simulink model "mic"  (Simulink 6.6)
libraries: mathlib x26, execlib x7, analoglib x4, genlib x3, arclib x1
settings Model: Creator=Student  LastModifiedBy=REX  MaskType=REX sequence  MaskIconFrame=on  MaskIconOpaque=on  MaskIconRotate=none  MaskIconUnits=autoscale

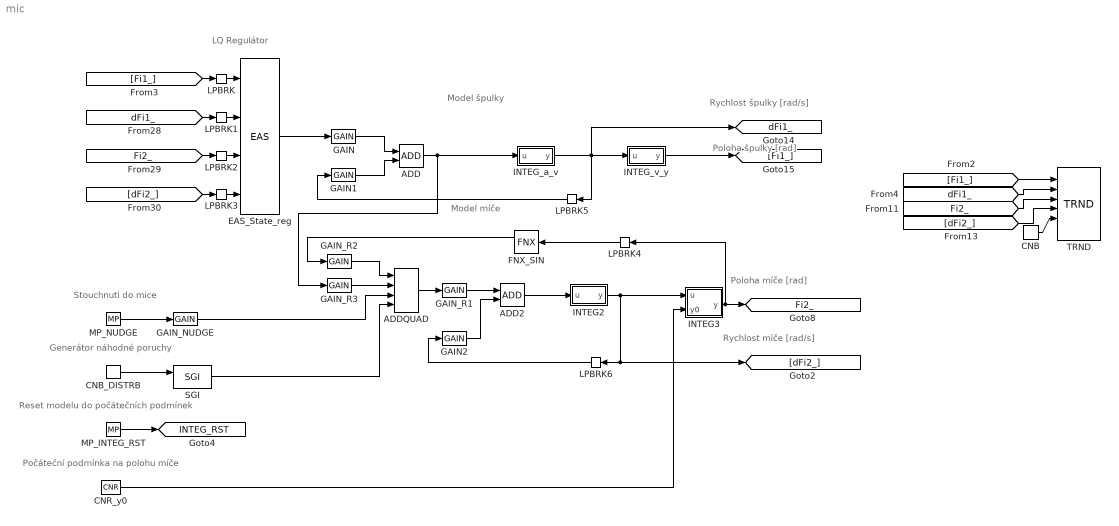
== system mic ==
  note: Stouchnuti do mice
  note: Generátor náhodné poruchy
  note: Reset modelu do počátečních podmínek
  note: Počáteční podmínka na polohu míče
  note: LQ Regulátor
  note: Rychlost špulky [rad/s]
  note: Poloha špulky [rad]
  note: Poloha míče [rad]
  note: Rychlost míče [rad/s]
  note: Model špulky
  note: Model míče
  ADD : mathlib/ADD
  ADD2 : mathlib/ADD
  ADDQUAD : mathlib/ADDQUAD  nl=0
  CNB : mathlib/CNB  SystemSampleTime=-1  YCN=on
  CNB_DISTRB : mathlib/CNB  SystemSampleTime=-1  YCN=on
  CNR_y0 : mathlib/CNR  ycn=0
  EAS_State_reg : mathlib/EAS  a=0.062399  b=1.26032  c=-45.7483  d=-6.60148  y0=0
  FNX_SIN : mathlib/FNX  Orientation=left  ifn=14: sin  yerr=0
  GAIN : mathlib/GAIN  k=85
  GAIN1 : mathlib/GAIN  k=-85
  GAIN2 : mathlib/GAIN  k=-0.3
  GAIN_NUDGE : mathlib/GAIN  k=-0.1
  GAIN_R1 : mathlib/GAIN  k=108.138
  GAIN_R2 : mathlib/GAIN  k=0.3994
  GAIN_R3 : mathlib/GAIN  k=0.0021
  INTEG2 : Subsystem
      mask Type: REX sequence
  INTEG3 : Subsystem
      mask Type: REX sequence
  INTEG_a_v : Subsystem
      mask Type: REX sequence
  INTEG_v_y : Subsystem
      mask Type: REX sequence
  LPBRK{,1..3} (4 alike) : execlib/LPBRK
  LPBRK4 : execlib/LPBRK  Orientation=left
  LPBRK5 : execlib/LPBRK  Orientation=left
  LPBRK6 : execlib/LPBRK  Orientation=left
  MP_INTEG_RST : genlib/MP  BSTATE=off  pwidth=0.5  RPTF=off
  MP_NUDGE : genlib/MP  BSTATE=on  pwidth=0.5  RPTF=off
  SGI : genlib/SGI  isig=4: RANDOM  amp=0.05  freq=1  phase=0  offset=0  ifrunit=1: Hz  iphunit=1: degrees
  TRND : arclib/TRND  SystemSampleTime=-1  n=4  l=10000  btype=8: Double  ptype1=1: Store  ptype2=1: Store  ptype3=1: Store  ptype4=1: Store  pfac=1  afac=0  arc=0  id=1  Title=Ball on spool  timesrc=1  ViewConfig="{\"View\":{\"Data\":{\"History\":20,\"XAxisTimeFormat\":66},\"PropertiesModel\":[{\"Id\":0,\"Items\":[{\"Color\":\"#000099\",\"Id\":0,\"IsActive\":true,\"LineWidth\":2,\"Name\":\"Fi1_\",\"SceneNumber\":1},{\"Color\":\"#669900\",\"Id\":1,\"IsActive\":true,\"LineWidth\":2,\"Name\":\"dFi1_\",\"SceneNumber\":2},{\"Color\":\"#ff0000\",\"Id\":2,\"IsActive\":true,\"LineWidth\":2,\"Name\":\"Fi2_\",\"SceneNumber\":1},{\"Color\":\"#9966cc\",\"Id\":3,\"IsActive\":true,\"LineWidth\":2,\"Name\":\"dFi2_\",\"SceneNumber\":3}]}],\"Scenes\":[{\"Id\":1},{\"Id\":2},{\"Id\":3}],\"sync\":false}}"
  tag scope: Fi2_=global, INTEG_RST=global, dFi1_=global
  wires:
  ADD/1 -> GAIN_R3/1, INTEG_a_v/1(u)
  ADD2/1 -> INTEG2/1(u)
  ADDQUAD/1 -> GAIN_R1/1
  CNB/1 -> TRND/5
  CNB_DISTRB/1 -> SGI/1
  CNR_y0/1 -> INTEG3/2(y0)
  EAS_State_reg/1 -> GAIN/1
  FNX_SIN/1 -> GAIN_R2/1
  [Fi2_] -> TRND/3
  [dFi2_] -> TRND/4
  [Fi1_] -> TRND/1
  [dFi1_] -> LPBRK1/1
  [Fi2_] -> LPBRK2/1
  [Fi1_] -> LPBRK/1
  [dFi2_] -> LPBRK3/1
  [dFi1_] -> TRND/2
  GAIN/1 -> ADD/1
  GAIN1/1 -> ADD/2
  GAIN2/1 -> ADD2/2
  GAIN_NUDGE/1 -> ADDQUAD/3
  GAIN_R1/1 -> ADD2/1
  GAIN_R2/1 -> ADDQUAD/1
  GAIN_R3/1 -> ADDQUAD/2
  INTEG2/1(y) -> [dFi2_], LPBRK6/1, INTEG3/1(u)
  INTEG3/1(y) -> [Fi2_], LPBRK4/1
  INTEG_a_v/1(y) -> [dFi1_], INTEG_v_y/1(u), LPBRK5/1
  INTEG_v_y/1(y) -> [Fi1_]
  LPBRK/1 -> EAS_State_reg/1
  LPBRK1/1 -> EAS_State_reg/2
  LPBRK2/1 -> EAS_State_reg/3
  LPBRK3/1 -> EAS_State_reg/4
  LPBRK4/1 -> FNX_SIN/1
  LPBRK5/1 -> GAIN1/1
  LPBRK6/1 -> GAIN2/1
  MP_INTEG_RST/1 -> [INTEG_RST]
  MP_NUDGE/1 -> GAIN_NUDGE/1
  SGI/1 -> ADDQUAD/4

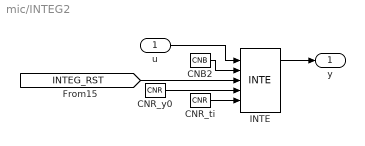
== system mic/INTEG2 ==
  u : Inport  Port=1  OutDataTypeStr=Inherit: auto
  CNB2 : mathlib/CNB  YCN=on
  CNR_ti : mathlib/CNR  ycn=1
  CNR_y0 : mathlib/CNR  ycn=0
  INTE : analoglib/INTE  ymin=-20  ymax=20
  y : Outport  Port=1  OutDataTypeStr=Inherit: auto
  wires:
  CNB2/1 -> INTE/2
  CNR_ti/1 -> INTE/5
  CNR_y0/1 -> INTE/4
  [INTEG_RST] -> INTE/3
  INTE/1 -> y/1
  u/1 -> INTE/1

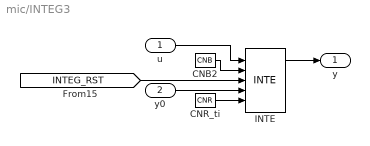
== system mic/INTEG3 ==
  u : Inport  Port=1  OutDataTypeStr=Inherit: auto
  y0 : Inport  Port=2  OutDataTypeStr=Inherit: auto
  CNB2 : mathlib/CNB  YCN=on
  CNR_ti : mathlib/CNR  ycn=1
  INTE : analoglib/INTE  ymin=-0.5  ymax=0.5
  y : Outport  Port=1  OutDataTypeStr=Inherit: auto
  wires:
  CNB2/1 -> INTE/2
  CNR_ti/1 -> INTE/5
  [INTEG_RST] -> INTE/3
  INTE/1 -> y/1
  u/1 -> INTE/1
  y0/1 -> INTE/4

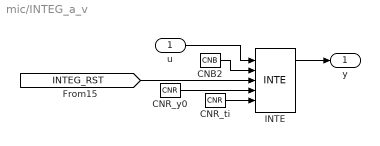
== system mic/INTEG_a_v ==
  u : Inport  Port=1  OutDataTypeStr=Inherit: auto
  CNB2 : mathlib/CNB  YCN=on
  CNR_ti : mathlib/CNR  ycn=1
  CNR_y0 : mathlib/CNR  ycn=0
  INTE : analoglib/INTE  ymin=-20  ymax=20
  y : Outport  Port=1  OutDataTypeStr=Inherit: auto
  wires:
  CNB2/1 -> INTE/2
  CNR_ti/1 -> INTE/5
  CNR_y0/1 -> INTE/4
  [INTEG_RST] -> INTE/3
  INTE/1 -> y/1
  u/1 -> INTE/1

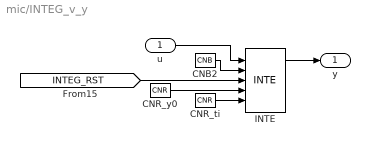
== system mic/INTEG_v_y ==
  u : Inport  Port=1  OutDataTypeStr=Inherit: auto
  CNB2 : mathlib/CNB  YCN=on
  CNR_ti : mathlib/CNR  ycn=1
  CNR_y0 : mathlib/CNR  ycn=0
  INTE : analoglib/INTE  ymin=-9999999999999999999999999999999999999  ymax=99999999999999999999999999999999999
  y : Outport  Port=1  OutDataTypeStr=Inherit: auto
  wires:
  CNB2/1 -> INTE/2
  CNR_ti/1 -> INTE/5
  CNR_y0/1 -> INTE/4
  [INTEG_RST] -> INTE/3
  INTE/1 -> y/1
  u/1 -> INTE/1
